simulink model "LVRT"  (R2019a)
settings: Solver=VariableStepAuto  StartTime=0.0  StopTime=5  RelTol=1e-3
libraries: powerlib_meascontrol x1
settings Model: Creator=sajid  LastModifiedBy=sajid

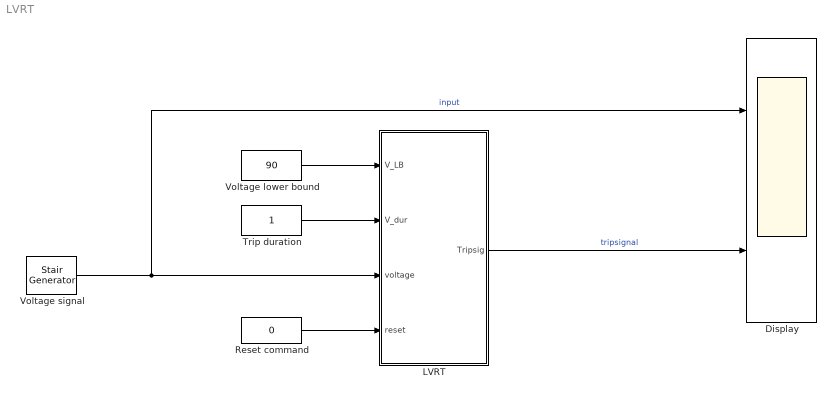
== system LVRT ==
  Display : Scope  NumInputPorts=2
  "LVRT " : Stateflow chart  BlockKeywords=__PRM__SERIALIZED__DATA__:Stateflow Chart,Stateflow Diagram  TreatAsAtomicUnit=on
  Reset command : Constant  Value=0
  Trip duration : Constant
  Voltage lower bound : Constant  Value=90
  "Voltage signal " : powerlib_meascontrol/Pulse & Signal Generators/Stair Generator  t=[0, 1,2,3,4,5]  e=[100,100,80,80,100,100]  Ts=0
      settings: SourceProductName=Simscape Electrical
  wires:
  "Voltage signal "/1 -> Display/1, "LVRT "/3(voltage)  "input"
  Reset command/1 -> "LVRT "/4(reset)
  "LVRT "/1(Tripsig) -> Display/2  "tripsignal"
  Voltage lower bound/1 -> "LVRT "/1(V_LB)
  Trip duration/1 -> "LVRT "/2(V_dur)

== stateflow chart LVRT/LVRT  ==
  state Normal
    Tripsig=0;
  state Trip
    Tripsig=1;
  (default) -> Normal
  Normal -> Trip : [duration(voltage<=V_LB)>V_dur]
  Trip -> Normal : [reset==1]
  data: V_LB input; V_dur input; Tripsig output; voltage input; reset input
